simulink model "doblependulo"  (R2022b)
settings: Solver=VariableStepAuto  StartTime=0.0  StopTime=10.0  MaxStep=0.0001  RelTol=1e-3
values from neighbouring files (symbols this model uses):
  g = 9.81    [parametros_doblependulo.m]
  l1 = 0.3    [parametros_doblependulo.m]
  l2 = 0.25    [parametros_doblependulo.m]
  m1 = 0.2    [parametros_doblependulo.m]
  m2 = 0.1    [parametros_doblependulo.m]
settings Model: Creator=Nestor  LastModifiedBy=Nestor

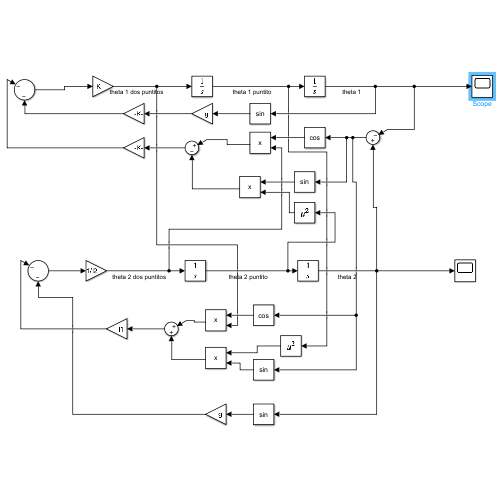
[thumbnail: Simulink's stored preview of the top-level diagram]
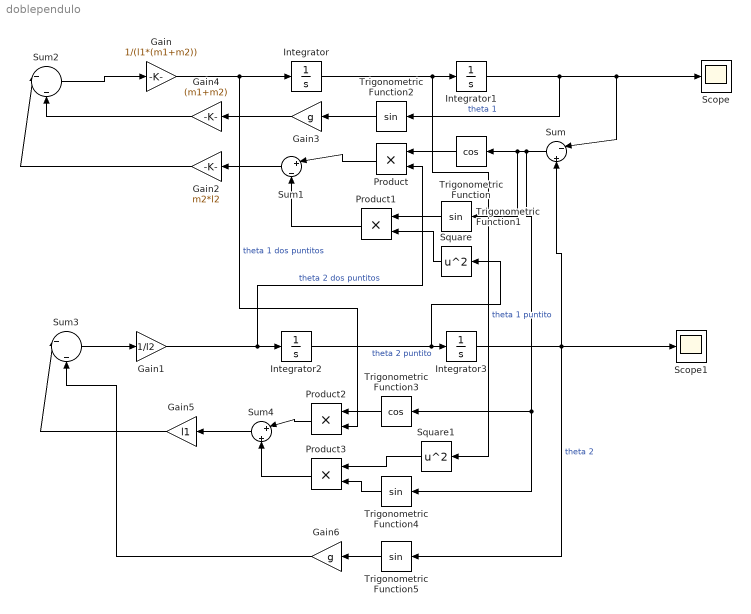
== system doblependulo ==
  Gain : Gain  Gain=1/(l1*(m1+m2))
  Gain1 : Gain  Gain=1/l2
  Gain2 : Gain  Gain=m2*l2
  Gain3 : Gain  Gain=g
  Gain4 : Gain  Gain=(m1+m2)
  Gain5 : Gain  Gain=l1
  Gain6 : Gain  Gain=g
  Integrator : Integrator
  Integrator1 : Integrator
  Integrator2 : Integrator
  Integrator3 : Integrator  InitialCondition=(35*pi)/180
  Product{,1..3} (4 alike) : Product
  Scope : Scope
  Scope1 : Scope
  Square : Math  Operator=square
  Square1 : Math  Operator=square
  Sum : Sum  Inputs=|-|+
  Sum1 : Sum  Inputs=|+|-
  Sum2 : Sum  Inputs=|-|-
  Sum3 : Sum  Inputs=|-|-
  Sum4 : Sum  Inputs=|+|+
  Trigonometric Function : Trigonometry  Operator=cos
  Trigonometric Function{1..2,4..5} (4 alike) : Trigonometry
  Trigonometric Function3 : Trigonometry  Operator=cos
  wires:
  Gain/1 -> Product2/2, Integrator/1  "theta 1 dos puntitos"
  Integrator/1 -> Square1/1, Integrator1/1  "theta 1 puntito"
  Integrator1/1 -> Trigonometric Function2/1, Scope/1, Sum/1  "theta 1"
  Gain1/1 -> Product/2, Integrator2/1  "theta 2 dos puntitos"
  Integrator3/1 -> Scope1/1, Trigonometric Function5/1, Sum/2  "theta 2"
  Integrator2/1 -> Square/1, Integrator3/1  "theta 2 puntito"
  Trigonometric Function/1 -> Product/1
  Product/1 -> Sum1/1
  Sum/1 -> Trigonometric Function4/1, Trigonometric Function3/1, Trigonometric Function1/1, Trigonometric Function/1
  Trigonometric Function1/1 -> Product1/1
  Square/1 -> Product1/2
  Product1/1 -> Sum1/2
  Sum1/1 -> Gain2/1
  Sum2/1 -> Gain/1
  Trigonometric Function2/1 -> Gain3/1
  Gain3/1 -> Gain4/1
  Gain4/1 -> Sum2/2
  Sum3/1 -> Gain1/1
  Trigonometric Function3/1 -> Product2/1
  Product2/1 -> Sum4/1
  Trigonometric Function4/1 -> Product3/2
  Square1/1 -> Product3/1
  Product3/1 -> Sum4/2
  Sum4/1 -> Gain5/1
  Trigonometric Function5/1 -> Gain6/1
  Gain6/1 -> Sum3/2
  Gain2/1 -> Sum2/1
  Gain5/1 -> Sum3/1
